simulink model "pendulum"  (R2025b)
settings: Solver=VariableStepAuto  StartTime=0.0  StopTime=30  RelTol=1e-3
InitFcn:
  | mass_sping_damper_init
values from neighbouring files (symbols this model uses):
  Kd = 0    [pendulum.m]
  Ki = 0    [pendulum.m]
  Kp = 0    [pendulum.m]
  N = 0    [pendulum.m]
settings Model: Creator=Muhammed E. Hamamci  LastModifiedBy=Muhammed E. Hamamci

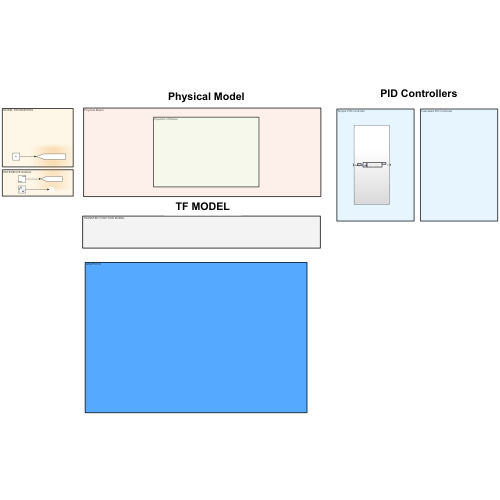
[thumbnail: Simulink's stored preview of the top-level diagram]
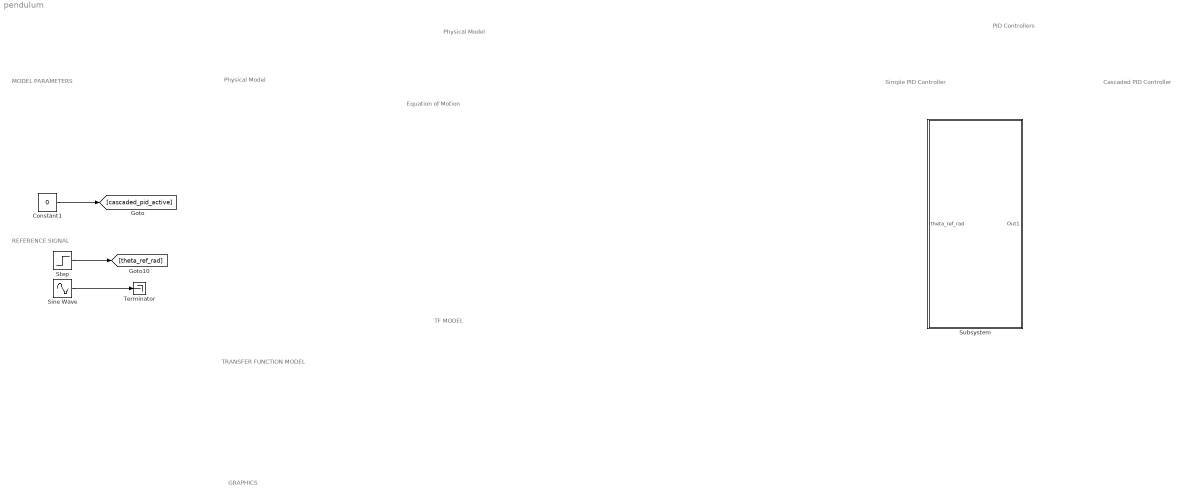
== system pendulum ==
  note: GRAPHICS
  note: TRANSFER FUNCTION MODEL
  note: Physical Model
  note: Physical Model
  note: Equation of Motion
  note: MODEL PARAMETERS
  note: TF MODEL
  note: PID Controllers
  note: Simple PID Controller
  note: REFERENCE SIGNAL
  note: Cascaded PID Controller
  Constant1 : Constant  Value=0
  Sine Wave : Sin  SampleTime=0
  Step : Step  SampleTime=0
  Subsystem : Subsystem
  Terminator : Terminator
  wires:
  Step/1 -> [theta_ref_rad]
  Sine Wave/1 -> Terminator/1
  Constant1/1 -> [cascaded_pid_active]

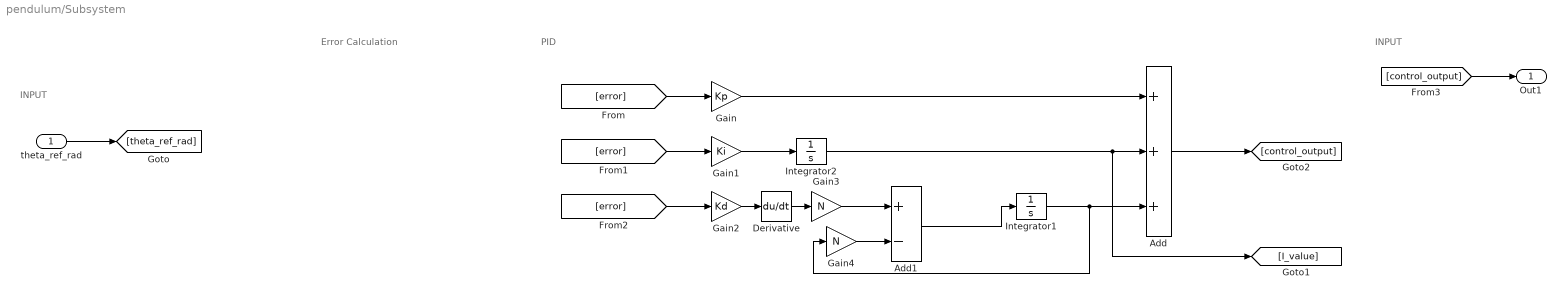
== system pendulum/Subsystem ==
  note: INPUT
  note: PID
  note: Error Calculation
  note: INPUT
  theta_ref_rad : Inport
  Add : Sum  Inputs=+++
  Add1 : Sum  Inputs=+-
  Derivative : Derivative
  Gain : Gain  Gain=Kp
  Gain1 : Gain  Gain=Ki
  Gain2 : Gain  Gain=Kd
  Gain3 : Gain  Gain=N
  Gain4 : Gain  Gain=N
  Integrator1 : Integrator
  Integrator2 : Integrator
  Out1 : Outport
  wires:
  theta_ref_rad/1 -> [theta_ref_rad]
  [error] -> Gain/1
  Integrator1/1 -> Gain4/1, Add/3
  Gain/1 -> Add/1
  Derivative/1 -> Gain3/1
  [error] -> Gain1/1
  Add/1 -> [control_output]
  Integrator2/1 -> [I_value], Add/2
  Gain2/1 -> Derivative/1
  Gain3/1 -> Add1/1
  Gain4/1 -> Add1/2
  [error] -> Gain2/1
  Gain1/1 -> Integrator2/1
  Add1/1 -> Integrator1/1
  [control_output] -> Out1/1
